simulink model "pdmMechanicalSystem"  (R2022a)
settings: Solver=FixedStepDiscrete  StartTime=0.0  StopTime=t(end)  FixedStep=Ts  RelTol=1e-3  EnableMultiTasking=on
PreLoadFcn:
  | Ts = 1/256;
  | t=(0:5120)'*Ts;
  | ynoi = 0.2;
  | groundnoi = 1;
  | PFnum = [0.00034    0.0017652   -0.0013829];
  | PFden = [1       -1.896      0.91629];
  | num0 = [1     -0.10075     -0.26052     -0.24022];
  | den0 = [1      -4.5049       8.2675      -7.7122       3.6508         -0.7];
  | numF = [1.2642     -0.12736     -0.32935     -0.30369];
  | denF = [1      -4.5674        8.511      -8.0697       3.8856     -0.75805];
  | den3 = (den0*0.25 + 0.75*denF);
  | num3 = (num0*0.25 + 0.75*numF);
  | seed = 1;
settings Model: Creator=The MathWorks, Inc.  LastModifiedBy=The MathWorks, Inc.
settings SolverCC: AlgebraicLoopSolver=TrustRegion  MinimalZcImpactIntegration=on
settings DataIOCC: LimitDataPoints=on  ReturnWorkspaceOutputs=off
settings OptimizationCC: LifeSpan=inf
settings DebuggingCC: UnconnectedInputMsg=warning  UnconnectedOutputMsg=warning  UnconnectedLineMsg=warning  AllowSymbolicDim=off  SFUnexpectedBacktrackingDiag=warning  SFNoUnconditionalDefaultTransitionDiag=warning  SFExecutionAtInitializationDiag=none  SFMachineParentedDataDiag=warning  ArithmeticOperatorsInVariantConditions=warning
settings HardwareCC: ProdBitPerPointer=32  ProdBitPerSizeT=32  ProdBitPerPtrDiffT=32  ProdLargestAtomicFloat=None  ProdIntDivRoundTo=Undefined  ProdEndianess=Unspecified  ProdWordSize=32  ProdHWDeviceType=32-bit Generic
settings ModelReferenceCC: PropagateSignalLabelsOutOfModel=off
settings SFSimCC: SimUseLocalCustomCode=off  CustomCodeUndefinedFunction=UseInterfaceOnly
settings RTWCC: RTWUseLocalCustomCode=off  DLArmComputeVersion=19.05
settings CodeAppCC: StateflowObjectComments=on
settings GRTTargetCC: TargetLangStandard=C89/C90 (ANSI)
settings ConfigComp: CovMetricSettings=dw  CovSaveCumulativeToWorkspaceVar=on  CovSaveSingleToWorkspaceVar=on  CovExternalEMLEnable=off

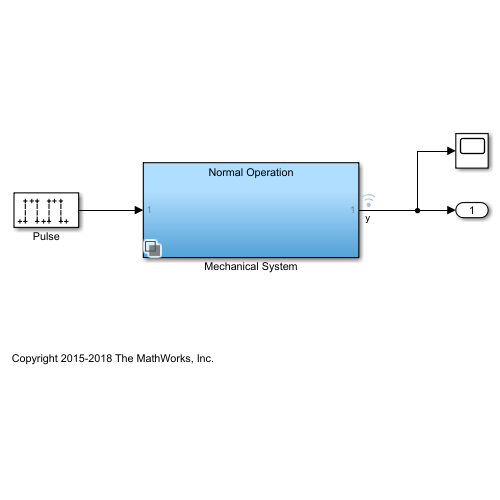
[thumbnail: Simulink's stored preview of the top-level diagram]
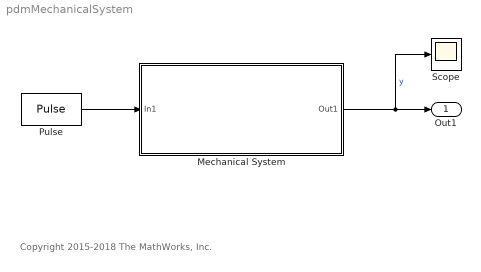
== system pdmMechanicalSystem ==
  note: Copyright 2015-2018 The MathWorks, Inc.
  Mechanical System : Subsystem  Variant=on  VariantControlMode=label  LabelModeActiveChoice=Normal
  Pulse : DiscretePulseGenerator  Amplitude=5  Period=512  SampleTime=Ts
  Scope : Scope
  Out1 : Outport  VectorParamsAs1DForOutWhenUnconnected=off
  wires:
  Pulse/1 -> Mechanical System/1(In1)
  Mechanical System/1(Out1) -> Scope/1, Out1/1  "y"

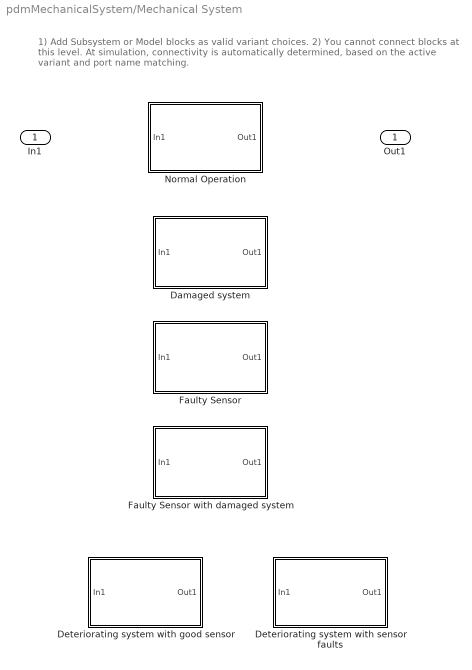
== system pdmMechanicalSystem/Mechanical System ==
  note: 1) Add Subsystem or Model blocks as valid variant choices.
      | 2) You cannot connect blocks at this level. At simulation, connectivity is automatically
      | determined, based on the active variant and port name matching.
  In1 : Inport
  Damaged system : Subsystem  VariantControl=DamagedSystem
  Deteriorating system with good sensor : Subsystem  VariantControl=DeterioratingSystem
  Deteriorating system with sensor faults : Subsystem  VariantControl=DeterioratingSystemFaultySensor
  Faulty Sensor : Subsystem  VariantControl=FaultySensor
  Faulty Sensor with damaged system : Subsystem  VariantControl=DamagedSystemFaultySensor
  Normal Operation : Subsystem  VariantControl=Normal
  Out1 : Outport  VectorParamsAs1DForOutWhenUnconnected=off

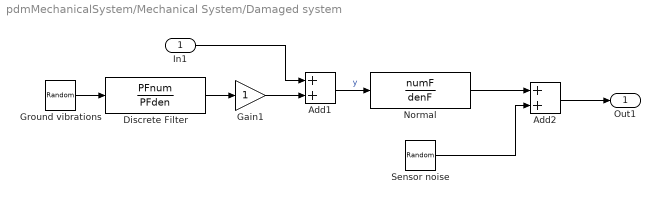
== system pdmMechanicalSystem/Mechanical System/Damaged system ==
  In1 : Inport
  Add1 : Sum
  Add2 : Sum
  Discrete Filter : DiscreteFilter  Numerator=PFnum  Denominator=PFden
  Gain1 : Gain
  Ground vibrations : RandomNumber  Variance=groundnoi  SampleTime=Ts
  Normal : DiscreteFilter  Numerator=numF  Denominator=denF
  Sensor noise : RandomNumber  Variance=ynoi  Seed=1  SampleTime=Ts
  Out1 : Outport  VectorParamsAs1DForOutWhenUnconnected=off
  wires:
  Discrete Filter/1 -> Gain1/1
  In1/1 -> Add1/1
  Gain1/1 -> Add1/2
  Add1/1 -> Normal/1  "y"
  Normal/1 -> Add2/1
  Sensor noise/1 -> Add2/2
  Add2/1 -> Out1/1
  Ground vibrations/1 -> Discrete Filter/1

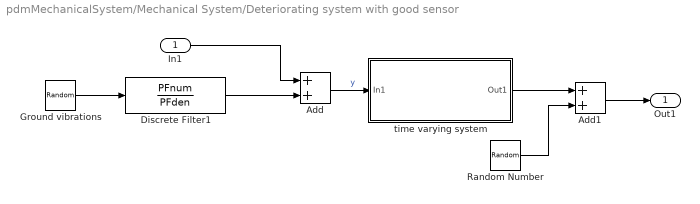
== system pdmMechanicalSystem/Mechanical System/Deteriorating system with good sensor ==
  In1 : Inport
  Add : Sum
  Add1 : Sum
  Discrete Filter1 : DiscreteFilter  Numerator=PFnum  Denominator=PFden
  Ground vibrations : RandomNumber  Variance=groundnoi  Seed=seed  SampleTime=Ts
  Random Number : RandomNumber  Variance=ynoi  SampleTime=Ts
  time varying system : Subsystem
  Out1 : Outport  VectorParamsAs1DForOutWhenUnconnected=off
  wires:
  In1/1 -> Add/1
  Discrete Filter1/1 -> Add/2
  Random Number/1 -> Add1/2
  Add1/1 -> Out1/1
  Ground vibrations/1 -> Discrete Filter1/1
  Add/1 -> time varying system/1(In1)  "y"
  time varying system/1(Out1) -> Add1/1

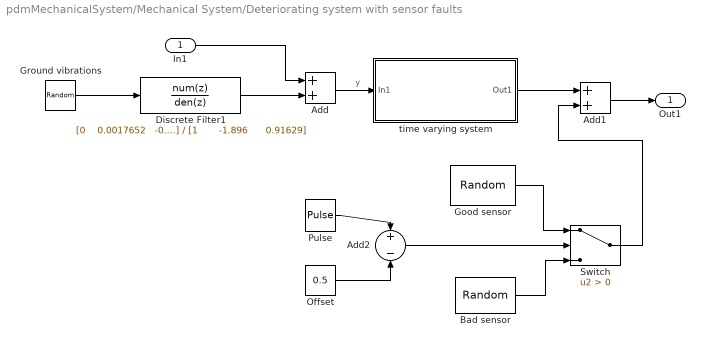
== system pdmMechanicalSystem/Mechanical System/Deteriorating system with sensor faults ==
  In1 : Inport
  Add : Sum
  Add1 : Sum
  Add2 : Sum  Inputs=+-
  Bad sensor : RandomNumber  Mean=.1  Variance=3  SampleTime=Ts
  Discrete Filter1 : DiscreteFilter  Numerator="[0    0.0017652   -0.0013829]"  Denominator="[1       -1.896      0.91629]"
  Good sensor : RandomNumber  Variance=ynoi  SampleTime=Ts
  Ground vibrations : RandomNumber  Variance=.5  SampleTime=Ts
  Offset : Constant  Value=0.5
  "Pulse " : DiscretePulseGenerator  Period=1024*12  PulseWidth=512*12  SampleTime=Ts
  Switch : Switch  Criteria=u2 > Threshold  SaturateOnIntegerOverflow=off  InputSameDT=off
  time varying system : Subsystem
  Out1 : Outport  VectorParamsAs1DForOutWhenUnconnected=off
  wires:
  In1/1 -> Add/1
  Discrete Filter1/1 -> Add/2
  Add1/1 -> Out1/1
  Add/1 -> time varying system/1(In1)  "y"
  time varying system/1(Out1) -> Add1/1
  "Pulse "/1 -> Add2/1
  Offset/1 -> Add2/2
  Add2/1 -> Switch/2
  Good sensor/1 -> Switch/1
  Bad sensor/1 -> Switch/3
  Switch/1 -> Add1/2
  Ground vibrations/1 -> Discrete Filter1/1

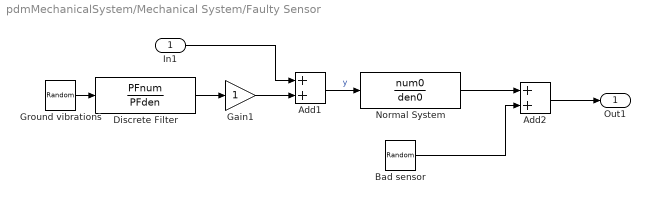
== system pdmMechanicalSystem/Mechanical System/Faulty Sensor ==
  In1 : Inport
  Add1 : Sum
  Add2 : Sum
  Bad sensor : RandomNumber  Mean=.1  Variance=3  SampleTime=Ts
  Discrete Filter : DiscreteFilter  Numerator=PFnum  Denominator=PFden
  Gain1 : Gain
  Ground vibrations : RandomNumber  Variance=groundnoi  SampleTime=Ts
  Normal System : DiscreteFilter  Numerator=num0  Denominator=den0
  Out1 : Outport  VectorParamsAs1DForOutWhenUnconnected=off
  wires:
  Discrete Filter/1 -> Gain1/1
  In1/1 -> Add1/1
  Gain1/1 -> Add1/2
  Add1/1 -> Normal System/1  "y"
  Normal System/1 -> Add2/1
  Bad sensor/1 -> Add2/2
  Add2/1 -> Out1/1
  Ground vibrations/1 -> Discrete Filter/1

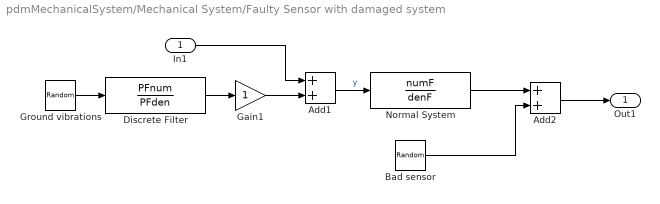
== system pdmMechanicalSystem/Mechanical System/Faulty Sensor with damaged system ==
  In1 : Inport
  Add1 : Sum
  Add2 : Sum
  Bad sensor : RandomNumber  Mean=.1  Variance=3  SampleTime=Ts
  Discrete Filter : DiscreteFilter  Numerator=PFnum  Denominator=PFden
  Gain1 : Gain
  Ground vibrations : RandomNumber  Variance=groundnoi  SampleTime=Ts
  Normal System : DiscreteFilter  Numerator=numF  Denominator=denF
  Out1 : Outport  VectorParamsAs1DForOutWhenUnconnected=off
  wires:
  Discrete Filter/1 -> Gain1/1
  In1/1 -> Add1/1
  Gain1/1 -> Add1/2
  Add1/1 -> Normal System/1  "y"
  Normal System/1 -> Add2/1
  Bad sensor/1 -> Add2/2
  Add2/1 -> Out1/1
  Ground vibrations/1 -> Discrete Filter/1

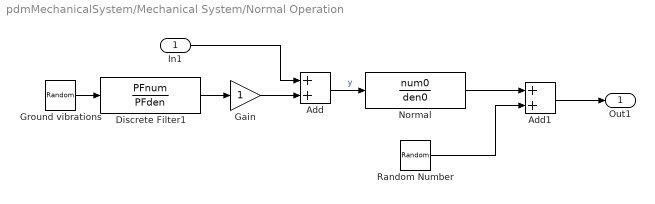
== system pdmMechanicalSystem/Mechanical System/Normal Operation ==
  In1 : Inport
  Add : Sum
  Add1 : Sum
  Discrete Filter1 : DiscreteFilter  Numerator=PFnum  Denominator=PFden
  Gain : Gain
  Ground vibrations : RandomNumber  Variance=groundnoi  SampleTime=Ts
  Normal : DiscreteFilter  Numerator=num0  Denominator=den0
  Random Number : RandomNumber  Variance=ynoi  SampleTime=Ts
  Out1 : Outport  VectorParamsAs1DForOutWhenUnconnected=off
  wires:
  Discrete Filter1/1 -> Gain/1
  In1/1 -> Add/1
  Gain/1 -> Add/2
  Add/1 -> Normal/1  "y"
  Normal/1 -> Add1/1
  Random Number/1 -> Add1/2
  Add1/1 -> Out1/1
  Ground vibrations/1 -> Discrete Filter1/1

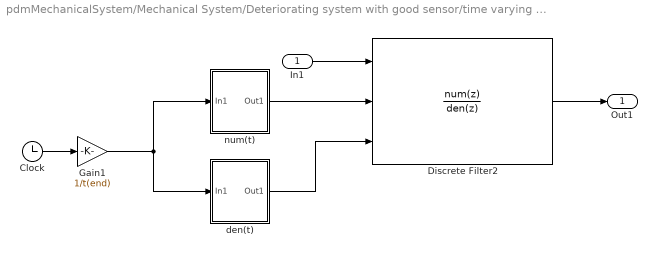
== system pdmMechanicalSystem/Mechanical System/Deteriorating system with good sensor/time varying system ==
  In1 : Inport
  Clock : Clock
  Discrete Filter2 : DiscreteFilter  NumeratorSource=Input port  Numerator=PFnum  DenominatorSource=Input port  Denominator=PFden  a0EqualsOne=on
      settings: InputPortMap=u0,p1,p3
  Gain1 : Gain  Gain=1/t(end)
  den(t) : Subsystem
  num(t) : Subsystem
  Out1 : Outport  VectorParamsAs1DForOutWhenUnconnected=off
  wires:
  Clock/1 -> Gain1/1
  Gain1/1 -> den(t)/1(In1), num(t)/1(In1)
  In1/1 -> Discrete Filter2/1
  Discrete Filter2/1 -> Out1/1
  num(t)/1(Out1) -> Discrete Filter2/2
  den(t)/1(Out1) -> Discrete Filter2/3

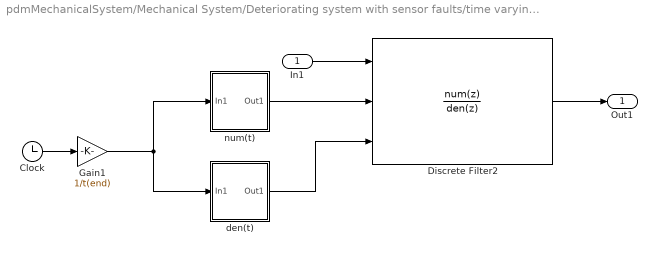
== system pdmMechanicalSystem/Mechanical System/Deteriorating system with sensor faults/time varying system ==
  In1 : Inport
  Clock : Clock
  Discrete Filter2 : DiscreteFilter  NumeratorSource=Input port  Numerator=PFnum  DenominatorSource=Input port  Denominator=PFden  a0EqualsOne=on
      settings: InputPortMap=u0,p1,p3
  Gain1 : Gain  Gain=1/t(end)
  den(t) : Subsystem
  num(t) : Subsystem
  Out1 : Outport  VectorParamsAs1DForOutWhenUnconnected=off
  wires:
  Clock/1 -> Gain1/1
  Gain1/1 -> den(t)/1(In1), num(t)/1(In1)
  In1/1 -> Discrete Filter2/1
  Discrete Filter2/1 -> Out1/1
  num(t)/1(Out1) -> Discrete Filter2/2
  den(t)/1(Out1) -> Discrete Filter2/3

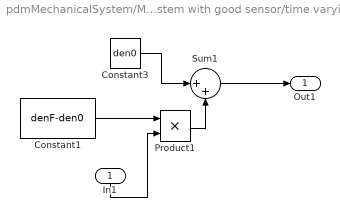
== system pdmMechanicalSystem/Mechanical System/Deteriorating system with good sensor/time varying system/den(t) ==
  In1 : Inport  SampleTime=Ts
  Constant1 : Constant  Value=denF-den0  SampleTime=Ts
  Constant3 : Constant  Value=den0  SampleTime=Ts
  Product1 : Product
  Sum1 : Sum  Inputs=|++
  Out1 : Outport  VectorParamsAs1DForOutWhenUnconnected=off
  wires:
  In1/1 -> Product1/2
  Sum1/1 -> Out1/1
  Constant3/1 -> Sum1/1
  Product1/1 -> Sum1/2
  Constant1/1 -> Product1/1

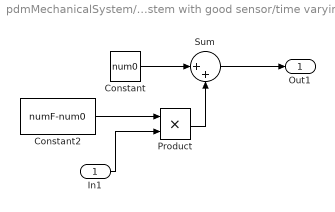
== system pdmMechanicalSystem/Mechanical System/Deteriorating system with good sensor/time varying system/num(t) ==
  In1 : Inport  SampleTime=Ts
  Constant : Constant  Value=num0  SampleTime=Ts
  Constant2 : Constant  Value=numF-num0  SampleTime=Ts
  Product : Product
  Sum : Sum  Inputs=|++
  Out1 : Outport  VectorParamsAs1DForOutWhenUnconnected=off
  wires:
  In1/1 -> Product/2
  Constant/1 -> Sum/1
  Sum/1 -> Out1/1
  Constant2/1 -> Product/1
  Product/1 -> Sum/2

== system pdmMechanicalSystem/Mechanical System/Deteriorating system with sensor faults/time varying system/den(t) ==
  In1 : Inport  SampleTime=Ts
  Constant1 : Constant  Value=denF-den0  SampleTime=Ts
  Constant3 : Constant  Value=den0  SampleTime=Ts
  Product1 : Product
  Sum1 : Sum  Inputs=|++
  Out1 : Outport  VectorParamsAs1DForOutWhenUnconnected=off
  wires:
  In1/1 -> Product1/2
  Sum1/1 -> Out1/1
  Constant3/1 -> Sum1/1
  Product1/1 -> Sum1/2
  Constant1/1 -> Product1/1

== system pdmMechanicalSystem/Mechanical System/Deteriorating system with sensor faults/time varying system/num(t) ==
  In1 : Inport  SampleTime=Ts
  Constant : Constant  Value=num0  SampleTime=Ts
  Constant2 : Constant  Value=numF-num0  SampleTime=Ts
  Product : Product
  Sum : Sum  Inputs=|++
  Out1 : Outport  VectorParamsAs1DForOutWhenUnconnected=off
  wires:
  In1/1 -> Product/2
  Constant/1 -> Sum/1
  Sum/1 -> Out1/1
  Constant2/1 -> Product/1
  Product/1 -> Sum/2
